simulink model "gearbox_sim"  (R2023b)
settings: Solver=VariableStepAuto  StartTime=0.0  StopTime=60  RelTol=1e-3
values from neighbouring files (symbols this model uses):
  A_f = 2.23    [init_params.m]    (also in matlab.mat)
  BSFC_min = 230    [matlab.mat]
  Crr = 0.012    [init_params.m]    (also in matlab.mat)
  Cx = 0.275    [init_params.m]    (also in matlab.mat)
  cycle_temps = [0 3 8 10 25 28 35 37 50 55 60]    [matlab.mat]
  cycle_vitesse = [0 2 5.56 5.56 5.56 5.56 13.9 13.9 13.9 5 0]    [matlab.mat]
  engine_rpm = [800 1500 2000 2500 3000 3500 4500 5500 6500]    [init_params.m]    (also in matlab.mat)
  engine_torque = [150 250  250  250  250  250  220  190  150]    [init_params.m]    (also in matlab.mat = [150 250 250 250 250 250 220 190 150])
  final_drive = 3.94    [init_params.m]    (also in matlab.mat)
  g = 9.81    [init_params.m]    (also in matlab.mat)
  m = 1310    [init_params.m]    (also in matlab.mat)
  r_w = 0.316    [init_params.m]    (also in matlab.mat)
  rads2rpm = 60/(2*pi)    (= 9.54929658551)    [init_params.m]    (also in matlab.mat)
  regime_optimal = 2500    [matlab.mat]
  rho = 1.225    [init_params.m]    (also in matlab.mat)
  rpm2rads = 2*pi/60    (= 0.10471975512)    [init_params.m]    (also in matlab.mat)
  slope = 0    [init_params.m]    (also in matlab.mat)
  v0 = 0    [init_params.m]    (also in matlab.mat)
libraries: simulink x3, slpidlib x1
settings Model: Creator=tahaf  LastModifiedBy=tahaf

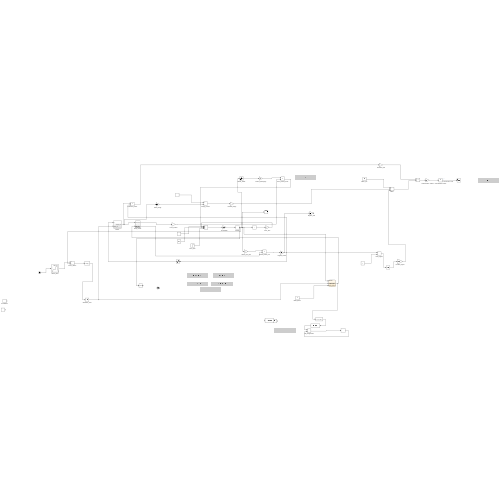
[thumbnail: Simulink's stored preview of the top-level diagram]
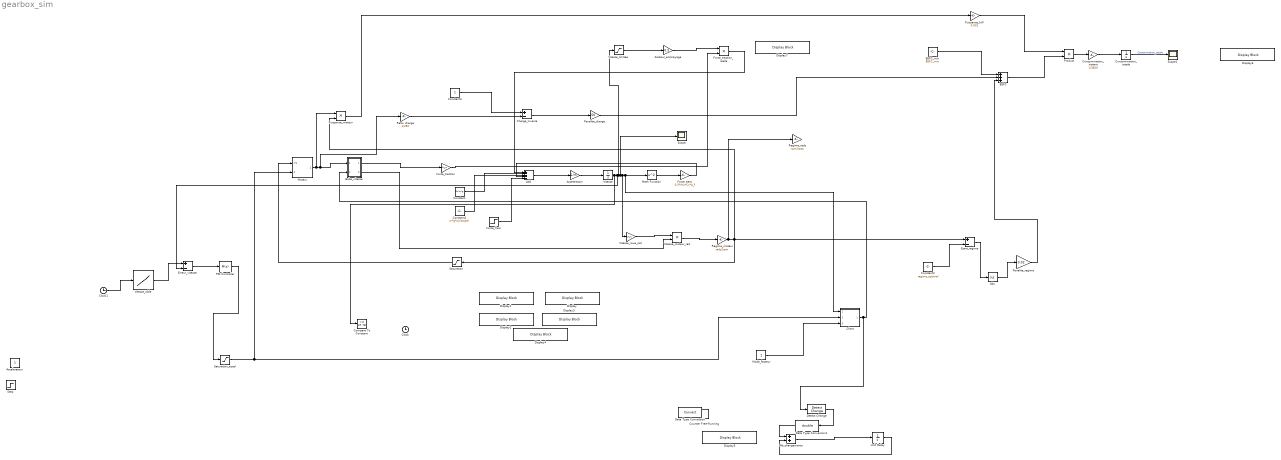
== system gearbox_sim ==
  Abs : Abs  SaturateOnIntegerOverflow=off
  Accelerateur : Constant
  Acceleration : Gain  Gain=1/m
  Add : Sum  Inputs=+----
  BSFC : Sum  Inputs=+++
  BSFC_min : Constant  Value=BSFC_min
  Boite_vitesse : Subsystem
  Charge_inverse : Sum  Inputs=+-
  Chart : Stateflow chart  TreatAsAtomicUnit=on
  Clock : Clock
  Clock1 : Clock
  Compare To Constant : simulink/Logic and Bit Operations/Compare To Constant  relop=>=  const=27.78  OutDataTypeStr=boolean
  Consommation_instant : Gain  Gain=1/3600
  Consommation_totale : Integrator
  Constant : Constant  Value=Crr*m*g
  Constant1 : Constant  Value=m*g*sin(slope)
  Constant2 : Constant  Value=regime_optimal
  Constant3 : Constant
  Counter Free-Running : simulink/Sources/Counter Free-Running  NumBits=16  tsamp=-1
  Data Type Conversion : DataTypeConversion  SaturateOnIntegerOverflow=off  RndMeth=Floor
  Data Type Conversion1 : DataTypeConversion  OutDataTypeStr=double  SaturateOnIntegerOverflow=off  RndMeth=Floor
  Detect Change : simulink/Logic and Bit Operations/Detect Change  vinit=1  OutDataTypeStr=boolean
  Display{,1..7} (8 alike) : DisplayBlock  LabelPosition=Hide  Transparency=1
  Ecart_regime : Sum  Inputs=+-
  Erreur_vitesse : Sum  Inputs=+-
  Facteur_embrayage : Gain  Gain=0.5
  Force_aero : Gain  Gain=0.5*rho*Cx*A_f
  Force_frein : Step  After=3000  SampleTime=0
  Force_traction : Gain  Gain=1/r_w
  Force_traction_reelle : Product
  Math Function : Math  Operator=square
  Mode_facteur : Constant
  Moteur : Subsystem
  Nb_changements : Sum
  PID Controller : slpidlib/PID Controller  Controller=PI  Form=Parallel  TimeDomain=Continuous-time  UseExternalTs=off  SampleTime=-1  IntegratorMethod=Forward Euler  FilterMethod=Forward Euler  ControllerParametersSource=internal  P=0.1  I=0.05  UseKiTs=off  D=0  N=100  UseFilter=on  TunerSelectOption=Transfer Function Based (PID Tuner App)  InitialConditionSource=internal  InitialConditionForIntegrator=0  InitialConditionForFilter=0  DifferentiatorICPrevScaledInput=0  ExternalReset=none  TrackingMode=off  Kt=1  LimitOutput=off  SatLimitsSource=internal  UpperSaturationLimit=inf  LowerSaturationLimit=-inf  LinearizeAsGain=on  AntiWindupMode=none  Kb=1  LimitIntegrator=off  UpperIntegratorSaturationLimit=inf  LowerIntegratorSaturationLimit=-inf  POutMin=[]  POutMax=[]  IOutMin=[]  IOutMax=[]  DOutMin=[]  DOutMax=[]  NOutMin=[]  NOutMax=[]  SumOutMin=[]  SumOutMax=[]  SaturationOutMin=[]  SaturationOutMax=[]  PParamMin=[]  PParamMax=[]  IParamMin=[]  IParamMax=[]  DParamMin=[]  DParamMax=[]  NParamMin=[]  NParamMax=[]  KbParamMin=[]  KbParamMax=[]  KtParamMin=[]  KtParamMax=[]  KbOutMin=[]  KbOutMax=[]  KtOutMin=[]  KtOutMax=[]  IntegratorOutMin=[]  IntegratorOutMax=[]  FilterOutMin=[]  FilterOutMax=[]  SumI1OutMin=[]  SumI1OutMax=[]  SumI2OutMin=[]  SumI2OutMax=[]  SumI3OutMin=[]  SumI3OutMax=[]  SumI4OutMin=[]  SumI4OutMax=[]  SumDOutMin=[]  SumDOutMax=[]  DifferentiatorOutMin=[]  DifferentiatorOutMax=[]  FilterDiffOutCoefMin=[]  FilterDiffOutCoefMax=[]  ReciprocalOutMin=[]  ReciprocalOutMax=[]  SumDenOutMin=[]  SumDenOutMax=[]  SumNumOutMin=[]  SumNumOutMax=[]  DivideOutMin=[]  DivideOutMax=[]  UdiffTsProdOutMin=[]  UdiffTsProdOutMax=[]  NTsProdOutMin=[]  NTsProdOutMax=[]  UintegralTsProdOutMin=[]  UintegralTsProdOutMax=[]  UngainTsProdOutMin=[]  UngainTsProdOutMax=[]  ClampingZeroOutDataTypeStr=Inherit: Inherit via back propagation  ClampingZeroOutMin=[]  ClampingZeroOutMax=[]  FilterDenConstantOutDataTypeStr=Inherit: Inherit via back propagation  FilterDenConstantOutMin=[]  FilterDenConstantOutMax=[]  PCopyOutDataTypeStr=Inherit: Inherit via back propagation  PCopyOutMin=[]  PCopyOutMax=[]  NCopyOutDataTypeStr=Inherit: Inherit via back propagation  NCopyOutMin=[]  NCopyOutMax=[]  IntegratorContinuousStateAttributes=''  IntegratorStateMustResolveToSignalObject=off  IntegratorRTWStateStorageClass=Auto  FilterContinuousStateAttributes=''  FilterStateMustResolveToSignalObject=off  FilterRTWStateStorageClass=Auto  ParallelPVariant=InternalParameters  IdealPVariant=Disabled  IVariant=InternalParameters  DVariant=Disabled  IntegratorVariant=Continuous  SatVariant=Disabled  AWVariant=Passthrough  PCopyVariant=Disabled  TRVariant=Disabled  FdbkBlocksVariant=Forward  IdealPFdbkVariant=Disabled  SatFdbkVariant=Disabled  DerivativeFilterVariant=Disabled  NVariant=Disabled  NCopyVariant=Disabled_SignalSpec  FilterICVariant=Disabled  IntegratorICVariant=InternalICs  ExternalResetVariant=Disabled  TRSumVariant=Passthrough  SumFdbkVariant=Disabled  SumVariant=Sum_PI  TsampFilterVariant=InternalTs  TsampNgainVariant=Passthrough  TsampIntegralVariant=Disabled_SignalSpec  ExternalSaturationOutDataTypeStr=Inherit: Same as second input
  Penalite_charge : Gain  Gain=50
  Penalite_regime : Gain  Gain=0.02
  Product : Product
  Puissance_kW : Gain  Gain=0.001
  Puissance_moteur : Product
  Ratio_charge : Gain  Gain=1/250
  Regime_moteur : Gain  Gain=rads2rpm
  Regime_rads : Gain  Gain=rpm2rads
  Saturation : Saturate  UpperLimit=6500  LowerLimit=800
  Saturation_accel : Saturate  UpperLimit=1  LowerLimit=0
  Scope : Scope
  Scope1 : Scope
  Step : Step  Time=5  Before=1  After=0  SampleTime=0
  Unit Delay : UnitDelay  SampleTime=-1  HasFrameUpgradeWarning=on
  Vitesse : Integrator  InitialCondition=v0
  Vitesse_cible : Lookup_n-D  NumberOfTableDimensions=1  BreakpointsForDimension1=cycle_temps  Table=cycle_vitesse  InternalRulePriority=Speed  RndMeth=Simplest
  Vitesse_limitee : Saturate  UpperLimit=2  LowerLimit=0.3
  Vitesse_moteur_rad : Product
  Vitesse_roue_rad : Gain  Gain=1/r_w
  wires:
  Boite_vitesse/1(Out1) -> Force_traction/1
  Force_traction/1 -> Force_traction_reelle/2
  Constant/1 -> Add/2
  Constant1/1 -> Add/3
  Add/1 -> Acceleration/1
  Acceleration/1 -> Vitesse/1
  Vitesse/1 -> Erreur_vitesse/2, Vitesse_limitee/1, Math Function/1, Chart/1(Vitesse), Vitesse_roue_rad/1, Scope/1, Compare To Constant/1
  Math Function/1 -> Force_aero/1
  Force_aero/1 -> Add/4
  Vitesse_roue_rad/1 -> Vitesse_moteur_rad/1
  Boite_vitesse/2(ratio_total) -> Vitesse_moteur_rad/2
  Vitesse_moteur_rad/1 -> Regime_moteur/1
  Regime_moteur/1 -> Regime_rads/1, Ecart_regime/1, Saturation/1, Puissance_moteur/2
  Saturation/1 -> Moteur/1(In1)
  Chart/1(rapport_actif) -> Detect Change/1, Boite_vitesse/2(rapport_actif)
  Moteur/1(couple_out) -> Puissance_moteur/1, Ratio_charge/1, Boite_vitesse/1(couple_out)
  Force_frein/1 -> Add/5
  Clock1/1 -> Vitesse_cible/1
  Vitesse_cible/1 -> Erreur_vitesse/1
  Saturation_accel/1 -> Moteur/2(accel_in), Chart/2(Accelerateur)
  Erreur_vitesse/1 -> PID Controller/1
  PID Controller/1 -> Saturation_accel/1
  Detect Change/1 -> Data Type Conversion1/1
  Nb_changements/1 -> Unit Delay/1
  Unit Delay/1 -> Nb_changements/2
  Data Type Conversion1/1 -> Nb_changements/1
  Mode_facteur/1 -> Chart/3(Mode_facteur)
  Constant2/1 -> Ecart_regime/2
  Ecart_regime/1 -> Abs/1
  Abs/1 -> Penalite_regime/1
  Constant3/1 -> Charge_inverse/1
  Ratio_charge/1 -> Charge_inverse/2
  Charge_inverse/1 -> Penalite_charge/1
  BSFC_min/1 -> BSFC/1
  Penalite_charge/1 -> BSFC/2
  Penalite_regime/1 -> BSFC/3
  Puissance_moteur/1 -> Puissance_kW/1
  Puissance_kW/1 -> Product/1
  BSFC/1 -> Product/2
  Product/1 -> Consommation_instant/1
  Consommation_instant/1 -> Consommation_totale/1
  Consommation_totale/1 -> Scope1/1  "Consommation_totale"
  Vitesse_limitee/1 -> Facteur_embrayage/1
  Facteur_embrayage/1 -> Force_traction_reelle/1
  Force_traction_reelle/1 -> Add/1

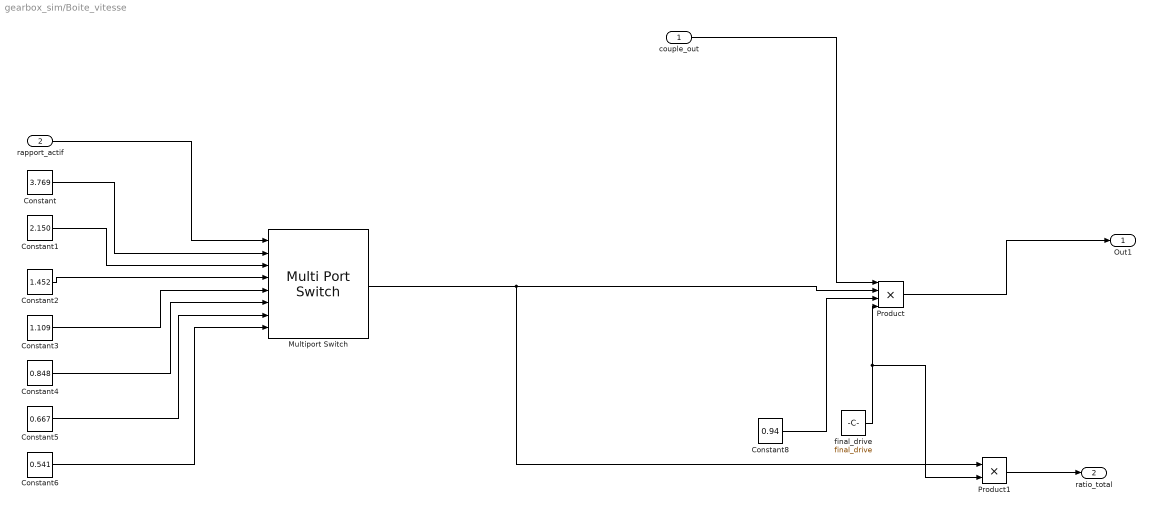
== system gearbox_sim/Boite_vitesse ==
  couple_out : Inport
  rapport_actif : Inport  Port=2
  Constant : Constant  Value=3.769
  Constant1 : Constant  Value=2.150
  Constant2 : Constant  Value=1.452
  Constant3 : Constant  Value=1.109
  Constant4 : Constant  Value=0.848
  Constant5 : Constant  Value=0.667
  Constant6 : Constant  Value=0.541
  Constant8 : Constant  Value=0.94
  Multiport Switch : MultiPortSwitch  Inputs=7  SaturateOnIntegerOverflow=off  InputSameDT=off
  Product : Product  Inputs=4
  Product1 : Product
  final_drive : Constant  Value=final_drive
  Out1 : Outport
  ratio_total : Outport  Port=2
  wires:
  Multiport Switch/1 -> Product1/1, Product/2
  Constant5/1 -> Multiport Switch/7
  Constant8/1 -> Product/3
  Constant/1 -> Multiport Switch/2
  Constant6/1 -> Multiport Switch/8
  Constant1/1 -> Multiport Switch/3
  Constant3/1 -> Multiport Switch/5
  Constant4/1 -> Multiport Switch/6
  Product/1 -> Out1/1
  Constant2/1 -> Multiport Switch/4
  couple_out/1 -> Product/1
  final_drive/1 -> Product1/2, Product/4
  Product1/1 -> ratio_total/1
  rapport_actif/1 -> Multiport Switch/1

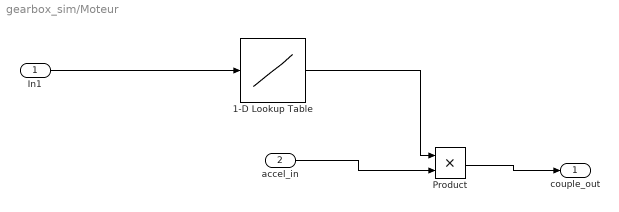
== system gearbox_sim/Moteur ==
  In1 : Inport
  accel_in : Inport  Port=2
  1-D Lookup Table : Lookup_n-D  NumberOfTableDimensions=1  BreakpointsForDimension1=engine_rpm  Table=engine_torque  InternalRulePriority=Speed  RndMeth=Simplest
  Product : Product
  couple_out : Outport
  wires:
  In1/1 -> 1-D Lookup Table/1
  1-D Lookup Table/1 -> Product/1
  accel_in/1 -> Product/2
  Product/1 -> couple_out/1

== stateflow chart gearbox_sim/Chart ==
  state Rapport1
    entry: rapport_actif = 1;
  state Rapport2
    entry: rapport_actif = 2;
  state Rapport3
    entry: rapport_actif = 3;
  state Rapport4
    entry: rapport_actif = 4;
  state Rapport5
    entry: rapport_actif = 5;
  state Rapport6
    entry: rapport_actif = 6;
  state Rapport7
    entry: rapport_actif = 7;
  Rapport2 -> Rapport1 [order 2] : [Vitesse < (3 + 2*Accelerateur)*Mode_facteur && after(1, sec)]
  Rapport3 -> Rapport2 [order 2] : [Vitesse < (8 + 4*Accelerateur)*Mode_facteur && after(1, sec)]
  Rapport4 -> Rapport3 [order 1] : [Vitesse < (17 + 10*Accelerateur)*Mode_facteur && after(1, sec)]
  (default) -> Rapport1
  Rapport1 -> Rapport2 : [Vitesse > (5 + 3*Accelerateur)*Mode_facteur && after(1, sec)]
  Rapport2 -> Rapport3 [order 1] : [Vitesse > (10 + 6*Accelerateur)*Mode_facteur && after(1, sec)]
  Rapport3 -> Rapport4 [order 1] : [Vitesse > (20 + 13*Accelerateur)*Mode_facteur  && after(1, sec)]
  Rapport4 -> Rapport5 [order 2] : [Vitesse > (30 + 20*Accelerateur)*Mode_facteur && after(1, sec)]
  Rapport5 -> Rapport4 [order 2] : [Vitesse < (26 + 15*Accelerateur)*Mode_facteur && after(1, sec)]
  Rapport5 -> Rapport6 [order 1] : [Vitesse > (45 + 20*Accelerateur)*Mode_facteur && after(1, sec)]
  Rapport6 -> Rapport7 [order 1] : [Vitesse > (60 + 25*Accelerateur)*Mode_facteur && after(1, sec)]
  Rapport6 -> Rapport5 [order 2] : [Vitesse < (40 + 18*Accelerateur)*Mode_facteur && after(1, sec)]
  Rapport7 -> Rapport6 : [Vitesse < (55 + 22*Accelerateur)*Mode_facteur && after(1, sec)]
  data: rapport_actif output; Vitesse input; Accelerateur input; Mode_facteur input
